simulink model "Sim_Modell_RFJ_2015b"  (R2015b)
settings: Solver=ode45  StartTime=0.0  StopTime=5  MaxStep=0.1  RelTol=1e-3
InitFcn:
  | Parameter_RFJ
undefined symbols (not defined in the file or in its folder): par_imp, par_reg
libraries: cstblocks x2, simulink x1
settings Model: Creator=ast  LastModifiedBy=danielhauer
settings DataIOCC: SaveFormat=Array  SignalLoggingSaveFormat=ModelDataLogs
settings OptimizationCC: ExpressionDepthLimit=2147483647  InitFltsAndDblsToZero=on
settings DebuggingCC: SaveWithParameterizedLinksMsg=none  UnderspecifiedInitializationDetection=Classic  MergeDetectMultiDrivingBlocksExec=none  SolverPrmCheckMsg=warning  MultiTaskDSMMsg=warning  MultiTaskCondExecSysMsg=none  FcnCallInpInsideContextMsg=UseLocalSettings  StateNameClashWarn=warning
settings HardwareCC: ProdBitPerPointer=32  ProdLargestAtomicFloat=None  ProdIntDivRoundTo=Undefined  ProdEndianess=Unspecified  ProdWordSize=32  ProdHWDeviceType=32-bit Generic
settings SFSimCC: SimParseCustomCode=off
settings GRTTargetCC: TargetFcnLib=ansi_tfl_tmw.mat  GeneratePreprocessorConditionals=Disable all  CombineOutputUpdateFcns=off  GRTInterface=on
settings ConfigComp: CovModelRefEnable=Off

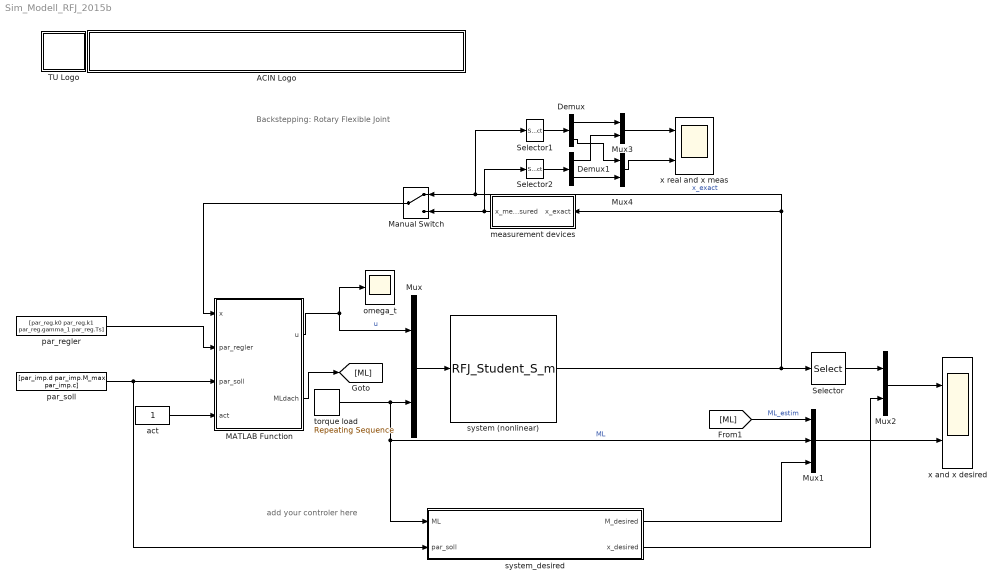
== system Sim_Modell_RFJ_2015b ==
  note: add your
      | controler
      | here
  note: Backstepping: Rotary Flexible Joint
  ACIN Logo : Subsystem
      mask init:
      | s = get_param(gcb,'UserData');
      mask Display:
      | image(s.logo,[0 0 439 45]);
      | %axis image
  Demux : Demux  Outputs=2
  Demux1 : Demux  Outputs=2
  MATLAB Function : MATLAB Function  TreatAsAtomicUnit=on
  Manual Switch : ManualSwitch
  Mux{,2..4} (4 alike) : Mux  Inputs=2
  Mux1 : Mux  Inputs=3
  Selector : Selector  InputPortWidth=3  IndexOptions=Index vector (dialog)  Indices=[1 2]  OutputSizes=1
  Selector1 : Selector  InputPortWidth=3  IndexOptions=Index vector (dialog)  Indices=[1 2]  OutputSizes=1
  Selector2 : Selector  InputPortWidth=3  IndexOptions=Index vector (dialog)  Indices=[1 2]  OutputSizes=1
  TU Logo : Subsystem
      mask init:
      | s = get_param(gcb,'UserData');
      mask Display: image(s.logo,[0 0 45 45]);
  act : Constant
  measurement devices : Subsystem
  omega_t : Scope
  par_regler : Constant  Value=[par_reg.k0 par_reg.k1 par_reg.gamma_1 par_reg.Ts]
  par_soll : Constant  Value=[par_imp.d par_imp.M_max par_imp.c]
  system (nonlinear) : M-S-Function  FunctionName=RFJ_Student_S_m
      mask init:
      | resources = get_param(gcb,'UserData');
      mask Display: image(resources.logo);
  system_desired : Subsystem
      mask init:
      | resources = get_param(gcb,'UserData');
      mask Display:
      | image(resources.logo);
      | port_label('output', 1, 'M_desired');
      | port_label('output', 2, 'x_desired');
      | port_label('input', 1, 'ML');
      | port_label('input', 2, 'par_soll');
  torque load : simulink/Sources/Repeating Sequence  rep_seq_t=[0 0.5 1 1.5 1.50001 5]  rep_seq_y=[0 0 1 1 0 0]*0.1
  x and x desired : Scope  NumInputPorts=2
  x real and x meas : Scope  NumInputPorts=2
  wires:
  MATLAB Function/1(u) -> Mux/1, omega_t/1  "u"
  torque load/1 -> Mux/2, Mux1/2, system_desired/1(ML)  "ML"
  system (nonlinear)/1 -> measurement devices/1(x_exact), Manual Switch/1, Selector1/1, Selector/1  "x_exact"
  [ML] -> Mux1/1  "ML_estim"
  measurement devices/1(x_measured) -> Manual Switch/2, Selector2/1
  Mux1/1 -> x and x desired/2
  par_regler/1 -> MATLAB Function/2(par_regler)
  Selector/1 -> Mux2/1
  Mux2/1 -> x and x desired/1
  system_desired/1(M_desired) -> Mux1/3
  system_desired/2(x_desired) -> Mux2/2
  Manual Switch/1 -> MATLAB Function/1(x)
  Selector1/1 -> Demux/1
  Selector2/1 -> Demux1/1
  Demux1/1 -> Mux3/2
  Demux/1 -> Mux3/1
  Mux3/1 -> x real and x meas/1
  Mux4/1 -> x real and x meas/2
  Demux1/2 -> Mux4/2
  Demux/2 -> Mux4/1
  Mux/1 -> system (nonlinear)/1
  par_soll/1 -> MATLAB Function/3(par_soll), system_desired/2(par_soll)
  act/1 -> MATLAB Function/4(act)
  MATLAB Function/2(MLdach) -> [ML]

== system Sim_Modell_RFJ_2015b/ACIN Logo ==

== system Sim_Modell_RFJ_2015b/TU Logo ==

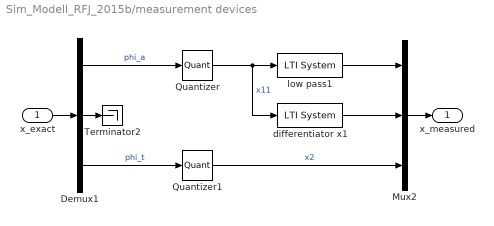
== system Sim_Modell_RFJ_2015b/measurement devices ==
  x_exact : Inport
  Demux1 : Demux  Outputs=3
  Mux2 : Mux  Inputs=3
  Quantizer : Quantizer  QuantizationInterval=2*pi/(3600*128)
  Quantizer1 : Quantizer  QuantizationInterval=2*pi/(2^16)
  Terminator2 : Terminator
  differentiator x1 : cstblocks/LTI System  sys=c2d( tf( [1 0], [1/500 1] ), 1e-3, 'foh')  IC=[]
  low pass1 : cstblocks/LTI System  sys=c2d( tf( [1], [1/500 1] ), 1e-3, 'zoh')  IC=[]
  x_measured : Outport
  wires:
  Demux1/3 -> Quantizer1/1  "phi_t"
  Demux1/1 -> Quantizer/1  "phi_a"
  Quantizer1/1 -> Mux2/3  "x2"
  Quantizer/1 -> low pass1/1, differentiator x1/1  "x11"
  Demux1/2 -> Terminator2/1
  x_exact/1 -> Demux1/1
  Mux2/1 -> x_measured/1
  differentiator x1/1 -> Mux2/2
  low pass1/1 -> Mux2/1

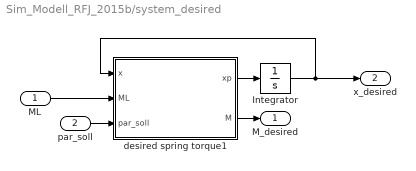
== system Sim_Modell_RFJ_2015b/system_desired ==
  ML : Inport
  par_soll : Inport  Port=2
  Integrator : Integrator  InitialCondition=[0 0]
  desired spring torque1 : MATLAB Function  TreatAsAtomicUnit=on
  M_desired : Outport
  x_desired : Outport  Port=2
  wires:
  desired spring torque1/1(xp) -> Integrator/1
  Integrator/1 -> desired spring torque1/1(x), x_desired/1
  ML/1 -> desired spring torque1/2(ML)
  desired spring torque1/2(M) -> M_desired/1
  par_soll/1 -> desired spring torque1/3(par_soll)

== matlab function Sim_Modell_RFJ_2015b/system_desired/desired spring torque1 ==
  data: x input; ML input; xp output; M output; par_soll input; par_sys parameter
function [xp, M] = fcn(x, ML, par_soll, par_sys)

% states
x11 = x(1);
x12 = x(2);  

% desired moment
M_max = par_soll(2);
c = par_soll(3);
M = M_max * tanh(c * x11 / M_max);

% desired damping
d = par_soll(1);

% desired positions
xp = zeros(2,1);
xp(1) = x12;
xp(2) = 1/par_sys.I_a * (ML - M - d*x12);

== matlab function Sim_Modell_RFJ_2015b/MATLAB Function ==
  settings: updateMethod=DISCRETE  sampleTime=par_reg.Ts
  data: x input; par_regler input; par_soll input; act input; u output; par_sys parameter; MLdach output
function [u,MLdach]   = Backstepping(x, par_regler, par_soll, act, par_sys)
% Implementierung eines wahnsinnig tollen Reglers
% inklusive herausragendem Lastmomentenschätzer

%% Parameter des Systems und des Reglers
persistent MLd;

if isempty(MLd)
    MLd=0;
end

k0      = par_regler(1);
k1      = par_regler(2); %k1 gewichtet x_2 - alpha(x_1) - siehe (3.24) im Laborskript
gamma_1 = par_regler(3);
Ts      = par_regler(4);

c0 = par_sys.c_0;
da = par_sys.d_a;
Ia = par_sys.I_a;

x_11 = x(1);
x_12 = x(2);
x_2  = x(3);

%% Soll-Parameter des Impedanz-Systems

d    = par_soll(1);
Mmax = par_soll(2);
c    = par_soll(3);


%% Regler und Schaetzer

if (act)
    
    M_x11=Mmax*tanh(c*x_11/Mmax);  
       
    u =  x_12 - x_12 / c0 * (1 - tanh(c * x_11 / Mmax) ^ 2)  * c + (da - d)/(Ia*c0) * (MLd - c0 * x_11+c0*x_2 - da * x_12) - 1 / gamma_1 * x_12 * c0 - k1 * (x_2 - x_11 + (M_x11 + (d - da) * x_12)/c0);

    MLd = MLd + k0 * Ts * ( x_2 - x_11 + ((d - da) * x_12 + M_x11 )/ c0)  *(d-da)/(c0*Ia);
     
else
    
    u = 0;

end

MLdach = MLd;

end
